simulink model "novo"  (R2025b)
settings: Solver=ode4  StartTime=0.0  StopTime=20  FixedStep=0.01  RelTol=1e-3
undefined symbols (not defined in the file): final_value, initial_value, step_time
libraries: cstblocks x5
settings Model: Creator=breno  LastModifiedBy=Breno

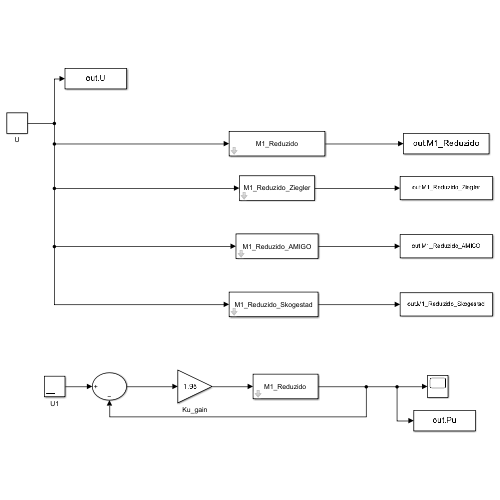
[thumbnail: Simulink's stored preview of the top-level diagram]
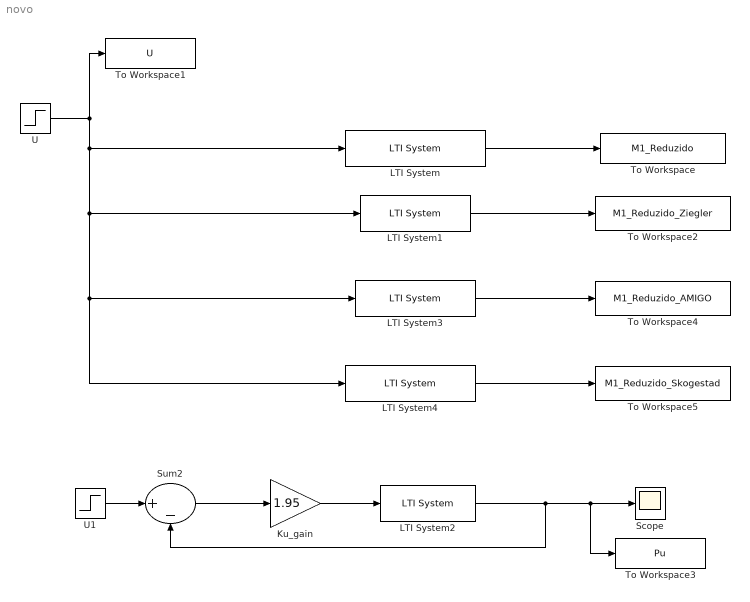
== system novo ==
  Ku_gain : Gain  Gain=1.95
  LTI System : cstblocks/LTI System  sys=M1_Reduzido  IC=[]  PadeOrder=0
  LTI System1 : cstblocks/LTI System  sys=M1_Reduzido_Ziegler  IC=[]  PadeOrder=0
  LTI System2 : cstblocks/LTI System  sys=M1_Reduzido  IC=[]  PadeOrder=0
  LTI System3 : cstblocks/LTI System  sys=M1_Reduzido_AMIGO  IC=[]  PadeOrder=0
  LTI System4 : cstblocks/LTI System  sys=M1_Reduzido_Skogestad  IC=[]  PadeOrder=0
  Scope : Scope
      settings: ActiveDisplayYMinimum=-2180.9644906891472  ActiveDisplayYMaximum=4779.0085246382705
  Sum2 : Sum  Inputs=|+-
  To Workspace : ToWorkspace  VariableName=M1_Reduzido  SaveFormat=Timeseries  SampleTime=-1
  To Workspace1 : ToWorkspace  VariableName=U  SaveFormat=Timeseries  SampleTime=-1
  To Workspace2 : ToWorkspace  VariableName=M1_Reduzido_Ziegler  SaveFormat=Timeseries  SampleTime=-1
  To Workspace3 : ToWorkspace  VariableName=Pu  SaveFormat=Timeseries  SampleTime=-1
  To Workspace4 : ToWorkspace  VariableName=M1_Reduzido_AMIGO  SaveFormat=Timeseries  SampleTime=-1
  To Workspace5 : ToWorkspace  VariableName=M1_Reduzido_Skogestad  SaveFormat=Timeseries  SampleTime=-1
  U : Step  Time=step_time  Before=initial_value  After=final_value  SampleTime=0
  U1 : Step  Time=step_time  Before=initial_value  After=final_value  SampleTime=0
  wires:
  Ku_gain/1 -> LTI System2/1
  Sum2/1 -> Ku_gain/1
  U1/1 -> Sum2/1
  LTI System2/1 -> Sum2/2, To Workspace3/1, Scope/1
  LTI System/1 -> To Workspace/1
  LTI System1/1 -> To Workspace2/1
  LTI System3/1 -> To Workspace4/1
  U/1 -> LTI System/1, LTI System1/1, LTI System3/1, LTI System4/1, To Workspace1/1
  LTI System4/1 -> To Workspace5/1
